simulink model "Automatisierung_subsystem"  (R2016b)
settings: Solver=ode1  StartTime=0.0  StopTime=Inf  FixedStep=0.001  RelTol=1e-3
PostLoadFcn:
  | , if any(exist('dsrtsu_mdlpostloadfcn', 'file') == [2, 3, 6]), try dsrtsu_mdlpostloadfcn('Execute', bdroot); catch fprintf('Error in PostLoadFcn (dsrtsu_mdlpostloadfcn) for model "%s":\n %s\n', bdroot, lasterr); end, end,
PreSaveFcn:
  | , if any(exist('dsmpb_private', 'file') == [2, 3, 6]), try, dsmpb_private('dsmpb_mdlclblib', 'PreSave', bdroot); catch, disp(lasterr); end, end,
CloseFcn:
  | , if any(exist('dsmpb_private', 'file') == [2, 3, 6]), try, dsmpb_private('dsmpb_mdlclblib', 'Close', bdroot); catch, disp(lasterr); end, end,
settings Model: DSRTSU_INTERNAL_RTI_VER=490  DSRTSU_INTERNAL_RTI_TYPE=rti1202  DSRTSU_INTERNAL_RTIFPGA=80  DSMPB_DATASERVER_ModelPortLibVersion1=8  DSMPB_DATASERVER_DataServerVersion1=6  DSMPB_DATASERVER_DataServerStreamVersion1=3  ParamWorkspaceSource=ReferencedWorkspace  Creator=verladebruecke  LastModifiedBy=Fritz
settings OptimizationCC: BlockReduction=off  OptimizeBlockIOStorage=off  BufferReuse=off  GlobalBufferReuse=off  ExpressionFolding=off  LocalBlockOutputs=off
settings HardwareCC: ProdBitPerPointer=32  ProdBitPerSizeT=32  ProdBitPerPtrDiffT=32  ProdLargestAtomicInteger=Integer  ProdEndianess=BigEndian  ProdWordSize=32  ProdHWDeviceType=Custom Processor->Custom  TargetIntDivRoundTo=Zero  TargetEndianess=BigEndian  TargetHWDeviceType=Custom Processor->Custom
settings RTWCC: SystemTargetFile=rti1202.tlc  MakeCommand=make_rti  TemplateMakefile=rti1202.tmf  Description=dSPACE DS1202 Hardware Platform
settings STFCustomTargetCC: ParMdlRefBuildCompliant=on  GRTInterface=off  SystemTargetFile=rti1202.tlc
settings GRTTargetCC: TargetLangStandard=C89/C90 (ANSI)  CompOptLevelCompliant=off  ConcurrentExecutionCompliant=off  CombineOutputUpdateFcns=off  MatFileLogging=off  CPPClassGenCompliant=off  UseToolchainInfoCompliant=off
settings ConfigComp: CovMetricSettings=dswe

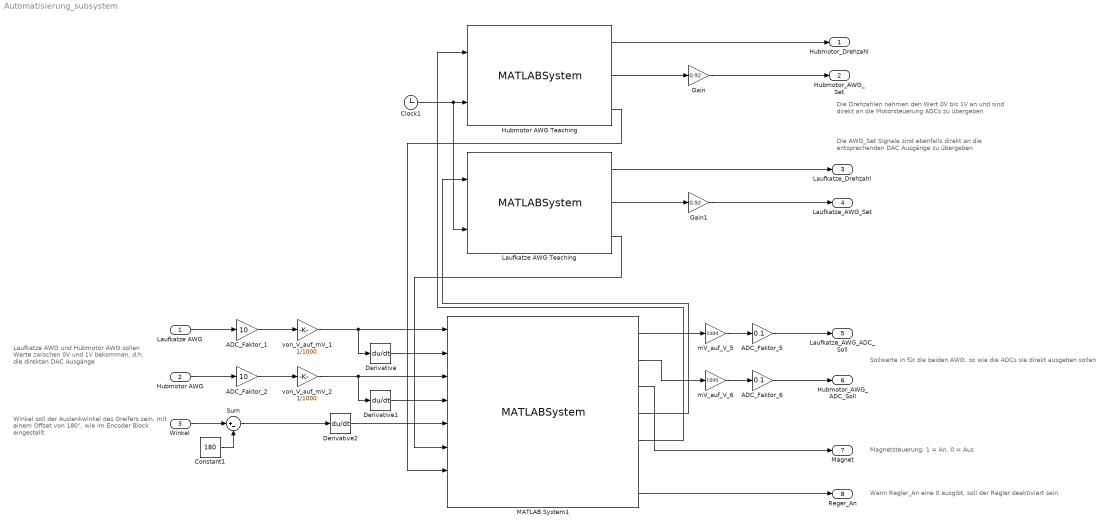
== system Automatisierung_subsystem ==
  note: Die AWG_Set Signale sind ebenfalls direkt an die
      | entsprechenden DAC Ausgänge zu übergeben
  note: Die Drehzahlen nehmen den Wert 0V bis 1V an und sind
      | direkt an die Motorsteuerung ADCs zu übergeben
  note: Magnetsteuerung: 1 = An, 0 = Aus
  note: Sollwerte in für die beiden AWG, so wie die ADCs sie direkt ausgeben sollen
  note: Wenn Regler_An eine 0 ausgibt, soll der Regler deaktiviert sein.
  note: Winkel soll der Auslenkwinkel des Greifers sein,
      | mit einem Offset von 180°, wie im
      | Encoder Block eingestellt
  note: Laufkatze AWG und Hubmotor AWG sollen
      | Werte zwischen 0V und 1V bekommen,
      | d.h. die direkten DAC Ausgänge
  Laufkatze AWG : Inport
  Hubmotor AWG : Inport  Port=2
  Winkel : Inport  Port=3
  ADC_Faktor_1 : Gain  Gain=10
  ADC_Faktor_2 : Gain  Gain=10
  ADC_Faktor_5 : Gain  Gain=0.1
  ADC_Faktor_6 : Gain  Gain=0.1
  Clock1 : Clock
  Constant1 : Constant  Value=180
  Derivative : Derivative
  Derivative1 : Derivative
  Derivative2 : Derivative
  Gain : Gain  Gain=0.92
  Gain1 : Gain  Gain=0.92
  Hubmotor AWG Teaching : MATLABSystem  System=Teaching  dauer_start_zu_endpunkt=40  motor_drehzahl=0.01  SimulateUsing=Code generation
      mask Type: Teaching
      mask Display:
      | disp('Teaching');
      | port_label('input',1,'Start');
      | port_label('input',2,'Clock');
      | port_label('output',1,'n_Motor');
      | port_label('output',2,'AWG_Set');
      | port_label('output',3,'Finished');
  Laufkatze AWG Teaching : MATLABSystem  System=Teaching  dauer_start_zu_endpunkt=40  motor_drehzahl=0.01  SimulateUsing=Code generation
      mask Type: Teaching
      mask Display:
      | disp('Teaching');
      | port_label('input',1,'Start');
      | port_label('input',2,'Clock');
      | port_label('output',1,'n_Motor');
      | port_label('output',2,'AWG_Set');
      | port_label('output',3,'Finished');
  MATLAB System1 : MATLABSystem  System=Steuerung_Automatisierung  box_sequence=[ 1, 2, 3, 4, 5 ]  needs_teaching=false  SimulateUsing=Code generation
      mask Type: Steuerung_Automatisierung
      mask Display:
      | disp('Steuerung_Automatisierung');
      | port_label('input',1,'horiz_value');
      | port_label('input',2,'horiz_speed');
      | port_label('input',3,'vert_value');
      | port_label('input',4,'vert_speed');
      | port_label('input',5,'angle_speed');
      | port_label('input',6,'horiz_teach_finished');
      | port_label('input',7,'vert_teach_finished');
      | port_label('input',8,'positioning_finished');
      | port_label('output',1,'horiz_setpoint');
      | port_label('output',2,'vert_setpoint');
      | port_label('output',3,'magnet_on');
      | port_label('output',4,'do_horiz_teach');
      | port_label('output',5,'do_vert_teach');
      | port_label('output',6,'do_positioning');
      | port_label('output',7,'control_enable');
  Sum : Sum  Inputs=|+-
  mV_auf_V_5 : Gain  Gain=1000
  mV_auf_V_6 : Gain  Gain=1000
  von_V_auf_mV_1 : Gain  Gain=1/1000
  von_V_auf_mV_2 : Gain  Gain=1/1000
  Hubmotor_Drehzahl : Outport
  Hubmotor_AWG_Set : Outport  Port=2
  Laufkatze_Drehzahl : Outport  Port=3
  Laufkatze_AWG_Set : Outport  Port=4
  Laufkatze_AWG_ADC_Soll : Outport  Port=5
  Hubmotor_AWG_ADC_Soll : Outport  Port=6
  Magnet : Outport  Port=7
  Reger_An : Outport  Port=8
  wires:
  Clock1/1 -> Laufkatze AWG Teaching/2, Hubmotor AWG Teaching/2
  Laufkatze AWG Teaching/3 -> MATLAB System1/6
  Hubmotor AWG Teaching/3 -> MATLAB System1/7
  MATLAB System1/4 -> Laufkatze AWG Teaching/1
  MATLAB System1/5 -> Hubmotor AWG Teaching/1
  Derivative/1 -> MATLAB System1/2
  Derivative1/1 -> MATLAB System1/4
  Derivative2/1 -> MATLAB System1/5
  von_V_auf_mV_1/1 -> Derivative/1, MATLAB System1/1
  Hubmotor AWG/1 -> ADC_Faktor_2/1
  von_V_auf_mV_2/1 -> Derivative1/1, MATLAB System1/3
  Constant1/1 -> Sum/2
  Winkel/1 -> Sum/1
  Sum/1 -> Derivative2/1
  Hubmotor AWG Teaching/1 -> Hubmotor_Drehzahl/1
  Laufkatze AWG Teaching/1 -> Laufkatze_Drehzahl/1
  MATLAB System1/1 -> mV_auf_V_5/1
  MATLAB System1/2 -> mV_auf_V_6/1
  MATLAB System1/3 -> Magnet/1
  MATLAB System1/7 -> Reger_An/1
  Gain/1 -> Hubmotor_AWG_Set/1
  Hubmotor AWG Teaching/2 -> Gain/1
  Gain1/1 -> Laufkatze_AWG_Set/1
  Laufkatze AWG Teaching/2 -> Gain1/1
  ADC_Faktor_2/1 -> von_V_auf_mV_2/1
  Laufkatze AWG/1 -> ADC_Faktor_1/1
  ADC_Faktor_1/1 -> von_V_auf_mV_1/1
  mV_auf_V_5/1 -> ADC_Faktor_5/1
  mV_auf_V_6/1 -> ADC_Faktor_6/1
  ADC_Faktor_6/1 -> Hubmotor_AWG_ADC_Soll/1
  ADC_Faktor_5/1 -> Laufkatze_AWG_ADC_Soll/1
